simulink model "pattern3x3_testing_2023v1"  (R2023a)
settings: Solver=FixedStepAuto  StartTime=0.0  StopTime=2  FixedStep=0.000005  RelTol=1e-3
values from neighbouring files (symbols this model uses):
  test_pattern = load('Pattern4_test.CSV')    [model_setup_test.m]
  Th_control_time2 = 0.02    [model_setup4.m]    (also in model_setup_test.m = 2)
  Th_minus_count2 = 10    [model_setup4.m]    (also in model_setup_test.m = 5)
  Th_plus_count2 = 20    [model_setup4.m]    (also in model_setup_test.m)
libraries: simulink x1
(part 2 of 4)

== system pattern3x3_testing_2023v1/Synapse12 ==
  note: Synapse
  Pre_spike : Inport
  addr : Inport  Port=2
  From Workspace : FromWorkspace  VariableName=syna_var
  MATLAB Function1 : MATLAB Function  TreatAsAtomicUnit=on
  Memory2 : Memory
  Product : Product
  Spike_gererator : Subsystem
  Weight : Outport
  Spike_out : Outport  Port=2
  Weight_out : Outport  Port=3
  wires:
  MATLAB Function1/1(y) -> Weight_out/1, Product/2
  Spike_gererator/1(Spike_out) -> Spike_out/1, Product/1
  Product/1 -> Weight/1
  Pre_spike/1 -> Memory2/1
  From Workspace/1 -> MATLAB Function1/1(syna_var)
  addr/1 -> MATLAB Function1/2(addr)
  Memory2/1 -> Spike_gererator/1("Spike ")

== system pattern3x3_testing_2023v1/Synapse13 ==
  note: Synapse
  Pre_spike : Inport
  addr : Inport  Port=2
  From Workspace : FromWorkspace  VariableName=syna_var
  MATLAB Function1 : MATLAB Function  TreatAsAtomicUnit=on
  Memory2 : Memory
  Product : Product
  Spike_gererator : Subsystem
  Weight : Outport
  Spike_out : Outport  Port=2
  Weight_out : Outport  Port=3
  wires:
  MATLAB Function1/1(y) -> Weight_out/1, Product/2
  Spike_gererator/1(Spike_out) -> Spike_out/1, Product/1
  Product/1 -> Weight/1
  Pre_spike/1 -> Memory2/1
  From Workspace/1 -> MATLAB Function1/1(syna_var)
  addr/1 -> MATLAB Function1/2(addr)
  Memory2/1 -> Spike_gererator/1("Spike ")

== system pattern3x3_testing_2023v1/Synapse14 ==
  note: Synapse
  Pre_spike : Inport
  addr : Inport  Port=2
  From Workspace : FromWorkspace  VariableName=syna_var
  MATLAB Function1 : MATLAB Function  TreatAsAtomicUnit=on
  Memory2 : Memory
  Product : Product
  Spike_gererator : Subsystem
  Weight : Outport
  Spike_out : Outport  Port=2
  Weight_out : Outport  Port=3
  wires:
  MATLAB Function1/1(y) -> Weight_out/1, Product/2
  Spike_gererator/1(Spike_out) -> Spike_out/1, Product/1
  Product/1 -> Weight/1
  Pre_spike/1 -> Memory2/1
  From Workspace/1 -> MATLAB Function1/1(syna_var)
  addr/1 -> MATLAB Function1/2(addr)
  Memory2/1 -> Spike_gererator/1("Spike ")

== system pattern3x3_testing_2023v1/Synapse15 ==
  note: Synapse
  Pre_spike : Inport
  addr : Inport  Port=2
  From Workspace : FromWorkspace  VariableName=syna_var
  MATLAB Function1 : MATLAB Function  TreatAsAtomicUnit=on
  Memory2 : Memory
  Product : Product
  Spike_gererator : Subsystem
  Weight : Outport
  Spike_out : Outport  Port=2
  Weight_out : Outport  Port=3
  wires:
  MATLAB Function1/1(y) -> Weight_out/1, Product/2
  Spike_gererator/1(Spike_out) -> Spike_out/1, Product/1
  Product/1 -> Weight/1
  Pre_spike/1 -> Memory2/1
  From Workspace/1 -> MATLAB Function1/1(syna_var)
  addr/1 -> MATLAB Function1/2(addr)
  Memory2/1 -> Spike_gererator/1("Spike ")

== system pattern3x3_testing_2023v1/Synapse16 ==
  note: Synapse
  Pre_spike : Inport
  addr : Inport  Port=2
  From Workspace : FromWorkspace  VariableName=syna_var
  MATLAB Function1 : MATLAB Function  TreatAsAtomicUnit=on
  Memory2 : Memory
  Product : Product
  Spike_gererator : Subsystem
  Weight : Outport
  Spike_out : Outport  Port=2
  Weight_out : Outport  Port=3
  wires:
  MATLAB Function1/1(y) -> Weight_out/1, Product/2
  Spike_gererator/1(Spike_out) -> Spike_out/1, Product/1
  Product/1 -> Weight/1
  Pre_spike/1 -> Memory2/1
  From Workspace/1 -> MATLAB Function1/1(syna_var)
  addr/1 -> MATLAB Function1/2(addr)
  Memory2/1 -> Spike_gererator/1("Spike ")

== system pattern3x3_testing_2023v1/Synapse17 ==
  note: Synapse
  Pre_spike : Inport
  addr : Inport  Port=2
  From Workspace : FromWorkspace  VariableName=syna_var
  MATLAB Function1 : MATLAB Function  TreatAsAtomicUnit=on
  Memory2 : Memory
  Product : Product
  Spike_gererator : Subsystem
  Weight : Outport
  Spike_out : Outport  Port=2
  Weight_out : Outport  Port=3
  wires:
  MATLAB Function1/1(y) -> Weight_out/1, Product/2
  Spike_gererator/1(Spike_out) -> Spike_out/1, Product/1
  Product/1 -> Weight/1
  Pre_spike/1 -> Memory2/1
  From Workspace/1 -> MATLAB Function1/1(syna_var)
  addr/1 -> MATLAB Function1/2(addr)
  Memory2/1 -> Spike_gererator/1("Spike ")

== system pattern3x3_testing_2023v1/Synapse18 ==
  note: Synapse
  Pre_spike : Inport
  addr : Inport  Port=2
  From Workspace : FromWorkspace  VariableName=syna_var
  MATLAB Function1 : MATLAB Function  TreatAsAtomicUnit=on
  Memory2 : Memory
  Product : Product
  Spike_gererator : Subsystem
  Weight : Outport
  Spike_out : Outport  Port=2
  Weight_out : Outport  Port=3
  wires:
  MATLAB Function1/1(y) -> Weight_out/1, Product/2
  Spike_gererator/1(Spike_out) -> Spike_out/1, Product/1
  Product/1 -> Weight/1
  Pre_spike/1 -> Memory2/1
  From Workspace/1 -> MATLAB Function1/1(syna_var)
  addr/1 -> MATLAB Function1/2(addr)
  Memory2/1 -> Spike_gererator/1("Spike ")

== system pattern3x3_testing_2023v1/Synapse19 ==
  note: Synapse
  Pre_spike : Inport
  addr : Inport  Port=2
  From Workspace : FromWorkspace  VariableName=syna_var
  MATLAB Function1 : MATLAB Function  TreatAsAtomicUnit=on
  Memory2 : Memory
  Product : Product
  Spike_gererator : Subsystem
  Weight : Outport
  Spike_out : Outport  Port=2
  Weight_out : Outport  Port=3
  wires:
  MATLAB Function1/1(y) -> Weight_out/1, Product/2
  Spike_gererator/1(Spike_out) -> Spike_out/1, Product/1
  Product/1 -> Weight/1
  Pre_spike/1 -> Memory2/1
  From Workspace/1 -> MATLAB Function1/1(syna_var)
  addr/1 -> MATLAB Function1/2(addr)
  Memory2/1 -> Spike_gererator/1("Spike ")

== system pattern3x3_testing_2023v1/Synapse2 ==
  note: Synapse
  Pre_spike : Inport
  addr : Inport  Port=2
  From Workspace : FromWorkspace  VariableName=syna_var
  MATLAB Function1 : MATLAB Function  TreatAsAtomicUnit=on
  Memory2 : Memory
  Product : Product
  Spike_gererator : Subsystem
  Weight : Outport
  Spike_out : Outport  Port=2
  Weight_out : Outport  Port=3
  wires:
  MATLAB Function1/1(y) -> Weight_out/1, Product/2
  Spike_gererator/1(Spike_out) -> Spike_out/1, Product/1
  Product/1 -> Weight/1
  Pre_spike/1 -> Memory2/1
  From Workspace/1 -> MATLAB Function1/1(syna_var)
  addr/1 -> MATLAB Function1/2(addr)
  Memory2/1 -> Spike_gererator/1("Spike ")

== system pattern3x3_testing_2023v1/Synapse20 ==
  note: Synapse
  Pre_spike : Inport
  addr : Inport  Port=2
  From Workspace : FromWorkspace  VariableName=syna_var
  MATLAB Function1 : MATLAB Function  TreatAsAtomicUnit=on
  Memory2 : Memory
  Product : Product
  Spike_gererator : Subsystem
  Weight : Outport
  Spike_out : Outport  Port=2
  Weight_out : Outport  Port=3
  wires:
  MATLAB Function1/1(y) -> Weight_out/1, Product/2
  Spike_gererator/1(Spike_out) -> Spike_out/1, Product/1
  Product/1 -> Weight/1
  Pre_spike/1 -> Memory2/1
  From Workspace/1 -> MATLAB Function1/1(syna_var)
  addr/1 -> MATLAB Function1/2(addr)
  Memory2/1 -> Spike_gererator/1("Spike ")

== system pattern3x3_testing_2023v1/Synapse21 ==
  note: Synapse
  Pre_spike : Inport
  addr : Inport  Port=2
  From Workspace : FromWorkspace  VariableName=syna_var
  MATLAB Function1 : MATLAB Function  TreatAsAtomicUnit=on
  Memory2 : Memory
  Product : Product
  Spike_gererator : Subsystem
  Weight : Outport
  Spike_out : Outport  Port=2
  Weight_out : Outport  Port=3
  wires:
  MATLAB Function1/1(y) -> Weight_out/1, Product/2
  Spike_gererator/1(Spike_out) -> Spike_out/1, Product/1
  Product/1 -> Weight/1
  Pre_spike/1 -> Memory2/1
  From Workspace/1 -> MATLAB Function1/1(syna_var)
  addr/1 -> MATLAB Function1/2(addr)
  Memory2/1 -> Spike_gererator/1("Spike ")

== system pattern3x3_testing_2023v1/Synapse22 ==
  note: Synapse
  Pre_spike : Inport
  addr : Inport  Port=2
  From Workspace : FromWorkspace  VariableName=syna_var
  MATLAB Function1 : MATLAB Function  TreatAsAtomicUnit=on
  Memory2 : Memory
  Product : Product
  Spike_gererator : Subsystem
  Weight : Outport
  Spike_out : Outport  Port=2
  Weight_out : Outport  Port=3
  wires:
  MATLAB Function1/1(y) -> Weight_out/1, Product/2
  Spike_gererator/1(Spike_out) -> Spike_out/1, Product/1
  Product/1 -> Weight/1
  Pre_spike/1 -> Memory2/1
  From Workspace/1 -> MATLAB Function1/1(syna_var)
  addr/1 -> MATLAB Function1/2(addr)
  Memory2/1 -> Spike_gererator/1("Spike ")

== system pattern3x3_testing_2023v1/Synapse23 ==
  note: Synapse
  Pre_spike : Inport
  addr : Inport  Port=2
  From Workspace : FromWorkspace  VariableName=syna_var
  MATLAB Function1 : MATLAB Function  TreatAsAtomicUnit=on
  Memory2 : Memory
  Product : Product
  Spike_gererator : Subsystem
  Weight : Outport
  Spike_out : Outport  Port=2
  Weight_out : Outport  Port=3
  wires:
  MATLAB Function1/1(y) -> Weight_out/1, Product/2
  Spike_gererator/1(Spike_out) -> Spike_out/1, Product/1
  Product/1 -> Weight/1
  Pre_spike/1 -> Memory2/1
  From Workspace/1 -> MATLAB Function1/1(syna_var)
  addr/1 -> MATLAB Function1/2(addr)
  Memory2/1 -> Spike_gererator/1("Spike ")

== system pattern3x3_testing_2023v1/Synapse24 ==
  note: Synapse
  Pre_spike : Inport
  addr : Inport  Port=2
  From Workspace : FromWorkspace  VariableName=syna_var
  MATLAB Function1 : MATLAB Function  TreatAsAtomicUnit=on
  Memory2 : Memory
  Product : Product
  Spike_gererator : Subsystem
  Weight : Outport
  Spike_out : Outport  Port=2
  Weight_out : Outport  Port=3
  wires:
  MATLAB Function1/1(y) -> Weight_out/1, Product/2
  Spike_gererator/1(Spike_out) -> Spike_out/1, Product/1
  Product/1 -> Weight/1
  Pre_spike/1 -> Memory2/1
  From Workspace/1 -> MATLAB Function1/1(syna_var)
  addr/1 -> MATLAB Function1/2(addr)
  Memory2/1 -> Spike_gererator/1("Spike ")

== system pattern3x3_testing_2023v1/Synapse25 ==
  note: Synapse
  Pre_spike : Inport
  addr : Inport  Port=2
  From Workspace : FromWorkspace  VariableName=syna_var
  MATLAB Function1 : MATLAB Function  TreatAsAtomicUnit=on
  Memory2 : Memory
  Product : Product
  Spike_gererator : Subsystem
  Weight : Outport
  Spike_out : Outport  Port=2
  Weight_out : Outport  Port=3
  wires:
  MATLAB Function1/1(y) -> Weight_out/1, Product/2
  Spike_gererator/1(Spike_out) -> Spike_out/1, Product/1
  Product/1 -> Weight/1
  Pre_spike/1 -> Memory2/1
  From Workspace/1 -> MATLAB Function1/1(syna_var)
  addr/1 -> MATLAB Function1/2(addr)
  Memory2/1 -> Spike_gererator/1("Spike ")

== system pattern3x3_testing_2023v1/Synapse26 ==
  note: Synapse
  Pre_spike : Inport
  addr : Inport  Port=2
  From Workspace : FromWorkspace  VariableName=syna_var
  MATLAB Function1 : MATLAB Function  TreatAsAtomicUnit=on
  Memory2 : Memory
  Product : Product
  Spike_gererator : Subsystem
  Weight : Outport
  Spike_out : Outport  Port=2
  Weight_out : Outport  Port=3
  wires:
  MATLAB Function1/1(y) -> Weight_out/1, Product/2
  Spike_gererator/1(Spike_out) -> Spike_out/1, Product/1
  Product/1 -> Weight/1
  Pre_spike/1 -> Memory2/1
  From Workspace/1 -> MATLAB Function1/1(syna_var)
  addr/1 -> MATLAB Function1/2(addr)
  Memory2/1 -> Spike_gererator/1("Spike ")

== system pattern3x3_testing_2023v1/Synapse27 ==
  note: Synapse
  Pre_spike : Inport
  addr : Inport  Port=2
  From Workspace : FromWorkspace  VariableName=syna_var
  MATLAB Function1 : MATLAB Function  TreatAsAtomicUnit=on
  Memory2 : Memory
  Product : Product
  Spike_gererator : Subsystem
  Weight : Outport
  Spike_out : Outport  Port=2
  Weight_out : Outport  Port=3
  wires:
  MATLAB Function1/1(y) -> Weight_out/1, Product/2
  Spike_gererator/1(Spike_out) -> Spike_out/1, Product/1
  Product/1 -> Weight/1
  Pre_spike/1 -> Memory2/1
  From Workspace/1 -> MATLAB Function1/1(syna_var)
  addr/1 -> MATLAB Function1/2(addr)
  Memory2/1 -> Spike_gererator/1("Spike ")

== system pattern3x3_testing_2023v1/Synapse28 ==
  note: Synapse
  Pre_spike : Inport
  addr : Inport  Port=2
  From Workspace : FromWorkspace  VariableName=syna_var
  MATLAB Function1 : MATLAB Function  TreatAsAtomicUnit=on
  Memory2 : Memory
  Product : Product
  Spike_gererator : Subsystem
  Weight : Outport
  Spike_out : Outport  Port=2
  Weight_out : Outport  Port=3
  wires:
  MATLAB Function1/1(y) -> Weight_out/1, Product/2
  Spike_gererator/1(Spike_out) -> Spike_out/1, Product/1
  Product/1 -> Weight/1
  Pre_spike/1 -> Memory2/1
  From Workspace/1 -> MATLAB Function1/1(syna_var)
  addr/1 -> MATLAB Function1/2(addr)
  Memory2/1 -> Spike_gererator/1("Spike ")

== system pattern3x3_testing_2023v1/Synapse29 ==
  note: Synapse
  Pre_spike : Inport
  addr : Inport  Port=2
  From Workspace : FromWorkspace  VariableName=syna_var
  MATLAB Function1 : MATLAB Function  TreatAsAtomicUnit=on
  Memory2 : Memory
  Product : Product
  Spike_gererator : Subsystem
  Weight : Outport
  Spike_out : Outport  Port=2
  Weight_out : Outport  Port=3
  wires:
  MATLAB Function1/1(y) -> Weight_out/1, Product/2
  Spike_gererator/1(Spike_out) -> Spike_out/1, Product/1
  Product/1 -> Weight/1
  Pre_spike/1 -> Memory2/1
  From Workspace/1 -> MATLAB Function1/1(syna_var)
  addr/1 -> MATLAB Function1/2(addr)
  Memory2/1 -> Spike_gererator/1("Spike ")

== system pattern3x3_testing_2023v1/Synapse3 ==
  note: Synapse
  Pre_spike : Inport
  addr : Inport  Port=2
  From Workspace : FromWorkspace  VariableName=syna_var
  MATLAB Function1 : MATLAB Function  TreatAsAtomicUnit=on
  Memory2 : Memory
  Product : Product
  Spike_gererator : Subsystem
  Weight : Outport
  Spike_out : Outport  Port=2
  Weight_out : Outport  Port=3
  wires:
  MATLAB Function1/1(y) -> Weight_out/1, Product/2
  Spike_gererator/1(Spike_out) -> Spike_out/1, Product/1
  Product/1 -> Weight/1
  Pre_spike/1 -> Memory2/1
  From Workspace/1 -> MATLAB Function1/1(syna_var)
  addr/1 -> MATLAB Function1/2(addr)
  Memory2/1 -> Spike_gererator/1("Spike ")

== system pattern3x3_testing_2023v1/Synapse30 ==
  note: Synapse
  Pre_spike : Inport
  addr : Inport  Port=2
  From Workspace : FromWorkspace  VariableName=syna_var
  MATLAB Function1 : MATLAB Function  TreatAsAtomicUnit=on
  Memory2 : Memory
  Product : Product
  Spike_gererator : Subsystem
  Weight : Outport
  Spike_out : Outport  Port=2
  Weight_out : Outport  Port=3
  wires:
  MATLAB Function1/1(y) -> Weight_out/1, Product/2
  Spike_gererator/1(Spike_out) -> Spike_out/1, Product/1
  Product/1 -> Weight/1
  Pre_spike/1 -> Memory2/1
  From Workspace/1 -> MATLAB Function1/1(syna_var)
  addr/1 -> MATLAB Function1/2(addr)
  Memory2/1 -> Spike_gererator/1("Spike ")

== system pattern3x3_testing_2023v1/Synapse31 ==
  note: Synapse
  Pre_spike : Inport
  addr : Inport  Port=2
  From Workspace : FromWorkspace  VariableName=syna_var
  MATLAB Function1 : MATLAB Function  TreatAsAtomicUnit=on
  Memory2 : Memory
  Product : Product
  Spike_gererator : Subsystem
  Weight : Outport
  Spike_out : Outport  Port=2
  Weight_out : Outport  Port=3
  wires:
  MATLAB Function1/1(y) -> Weight_out/1, Product/2
  Spike_gererator/1(Spike_out) -> Spike_out/1, Product/1
  Product/1 -> Weight/1
  Pre_spike/1 -> Memory2/1
  From Workspace/1 -> MATLAB Function1/1(syna_var)
  addr/1 -> MATLAB Function1/2(addr)
  Memory2/1 -> Spike_gererator/1("Spike ")

== system pattern3x3_testing_2023v1/Synapse32 ==
  note: Synapse
  Pre_spike : Inport
  addr : Inport  Port=2
  From Workspace : FromWorkspace  VariableName=syna_var
  MATLAB Function1 : MATLAB Function  TreatAsAtomicUnit=on
  Memory2 : Memory
  Product : Product
  Spike_gererator : Subsystem
  Weight : Outport
  Spike_out : Outport  Port=2
  Weight_out : Outport  Port=3
  wires:
  MATLAB Function1/1(y) -> Weight_out/1, Product/2
  Spike_gererator/1(Spike_out) -> Spike_out/1, Product/1
  Product/1 -> Weight/1
  Pre_spike/1 -> Memory2/1
  From Workspace/1 -> MATLAB Function1/1(syna_var)
  addr/1 -> MATLAB Function1/2(addr)
  Memory2/1 -> Spike_gererator/1("Spike ")

== system pattern3x3_testing_2023v1/Synapse33 ==
  note: Synapse
  Pre_spike : Inport
  addr : Inport  Port=2
  From Workspace : FromWorkspace  VariableName=syna_var
  MATLAB Function1 : MATLAB Function  TreatAsAtomicUnit=on
  Memory2 : Memory
  Product : Product
  Spike_gererator : Subsystem
  Weight : Outport
  Spike_out : Outport  Port=2
  Weight_out : Outport  Port=3
  wires:
  MATLAB Function1/1(y) -> Weight_out/1, Product/2
  Spike_gererator/1(Spike_out) -> Spike_out/1, Product/1
  Product/1 -> Weight/1
  Pre_spike/1 -> Memory2/1
  From Workspace/1 -> MATLAB Function1/1(syna_var)
  addr/1 -> MATLAB Function1/2(addr)
  Memory2/1 -> Spike_gererator/1("Spike ")

== system pattern3x3_testing_2023v1/Synapse34 ==
  note: Synapse
  Pre_spike : Inport
  addr : Inport  Port=2
  From Workspace : FromWorkspace  VariableName=syna_var
  MATLAB Function1 : MATLAB Function  TreatAsAtomicUnit=on
  Memory2 : Memory
  Product : Product
  Spike_gererator : Subsystem
  Weight : Outport
  Spike_out : Outport  Port=2
  Weight_out : Outport  Port=3
  wires:
  MATLAB Function1/1(y) -> Weight_out/1, Product/2
  Spike_gererator/1(Spike_out) -> Spike_out/1, Product/1
  Product/1 -> Weight/1
  Pre_spike/1 -> Memory2/1
  From Workspace/1 -> MATLAB Function1/1(syna_var)
  addr/1 -> MATLAB Function1/2(addr)
  Memory2/1 -> Spike_gererator/1("Spike ")

== system pattern3x3_testing_2023v1/Synapse35 ==
  note: Synapse
  Pre_spike : Inport
  addr : Inport  Port=2
  From Workspace : FromWorkspace  VariableName=syna_var
  MATLAB Function1 : MATLAB Function  TreatAsAtomicUnit=on
  Memory2 : Memory
  Product : Product
  Spike_gererator : Subsystem
  Weight : Outport
  Spike_out : Outport  Port=2
  Weight_out : Outport  Port=3
  wires:
  MATLAB Function1/1(y) -> Weight_out/1, Product/2
  Spike_gererator/1(Spike_out) -> Spike_out/1, Product/1
  Product/1 -> Weight/1
  Pre_spike/1 -> Memory2/1
  From Workspace/1 -> MATLAB Function1/1(syna_var)
  addr/1 -> MATLAB Function1/2(addr)
  Memory2/1 -> Spike_gererator/1("Spike ")

== system pattern3x3_testing_2023v1/Synapse36 ==
  note: Synapse
  Pre_spike : Inport
  addr : Inport  Port=2
  From Workspace : FromWorkspace  VariableName=syna_var
  MATLAB Function1 : MATLAB Function  TreatAsAtomicUnit=on
  Memory2 : Memory
  Product : Product
  Spike_gererator : Subsystem
  Weight : Outport
  Spike_out : Outport  Port=2
  Weight_out : Outport  Port=3
  wires:
  MATLAB Function1/1(y) -> Weight_out/1, Product/2
  Spike_gererator/1(Spike_out) -> Spike_out/1, Product/1
  Product/1 -> Weight/1
  Pre_spike/1 -> Memory2/1
  From Workspace/1 -> MATLAB Function1/1(syna_var)
  addr/1 -> MATLAB Function1/2(addr)
  Memory2/1 -> Spike_gererator/1("Spike ")

== system pattern3x3_testing_2023v1/Synapse4 ==
  note: Synapse
  Pre_spike : Inport
  addr : Inport  Port=2
  From Workspace : FromWorkspace  VariableName=syna_var
  MATLAB Function1 : MATLAB Function  TreatAsAtomicUnit=on
  Memory2 : Memory
  Product : Product
  Spike_gererator : Subsystem
  Weight : Outport
  Spike_out : Outport  Port=2
  Weight_out : Outport  Port=3
  wires:
  MATLAB Function1/1(y) -> Weight_out/1, Product/2
  Spike_gererator/1(Spike_out) -> Spike_out/1, Product/1
  Product/1 -> Weight/1
  Pre_spike/1 -> Memory2/1
  From Workspace/1 -> MATLAB Function1/1(syna_var)
  addr/1 -> MATLAB Function1/2(addr)
  Memory2/1 -> Spike_gererator/1("Spike ")

== system pattern3x3_testing_2023v1/Synapse5 ==
  note: Synapse
  Pre_spike : Inport
  addr : Inport  Port=2
  From Workspace : FromWorkspace  VariableName=syna_var
  MATLAB Function1 : MATLAB Function  TreatAsAtomicUnit=on
  Memory2 : Memory
  Product : Product
  Spike_gererator : Subsystem
  Weight : Outport
  Spike_out : Outport  Port=2
  Weight_out : Outport  Port=3
  wires:
  MATLAB Function1/1(y) -> Weight_out/1, Product/2
  Spike_gererator/1(Spike_out) -> Spike_out/1, Product/1
  Product/1 -> Weight/1
  Pre_spike/1 -> Memory2/1
  From Workspace/1 -> MATLAB Function1/1(syna_var)
  addr/1 -> MATLAB Function1/2(addr)
  Memory2/1 -> Spike_gererator/1("Spike ")

== system pattern3x3_testing_2023v1/Synapse6 ==
  note: Synapse
  Pre_spike : Inport
  addr : Inport  Port=2
  From Workspace : FromWorkspace  VariableName=syna_var
  MATLAB Function1 : MATLAB Function  TreatAsAtomicUnit=on
  Memory2 : Memory
  Product : Product
  Spike_gererator : Subsystem
  Weight : Outport
  Spike_out : Outport  Port=2
  Weight_out : Outport  Port=3
  wires:
  MATLAB Function1/1(y) -> Weight_out/1, Product/2
  Spike_gererator/1(Spike_out) -> Spike_out/1, Product/1
  Product/1 -> Weight/1
  Pre_spike/1 -> Memory2/1
  From Workspace/1 -> MATLAB Function1/1(syna_var)
  addr/1 -> MATLAB Function1/2(addr)
  Memory2/1 -> Spike_gererator/1("Spike ")

== system pattern3x3_testing_2023v1/Synapse7 ==
  note: Synapse
  Pre_spike : Inport
  addr : Inport  Port=2
  From Workspace : FromWorkspace  VariableName=syna_var
  MATLAB Function1 : MATLAB Function  TreatAsAtomicUnit=on
  Memory2 : Memory
  Product : Product
  Spike_gererator : Subsystem
  Weight : Outport
  Spike_out : Outport  Port=2
  Weight_out : Outport  Port=3
  wires:
  MATLAB Function1/1(y) -> Weight_out/1, Product/2
  Spike_gererator/1(Spike_out) -> Spike_out/1, Product/1
  Product/1 -> Weight/1
  Pre_spike/1 -> Memory2/1
  From Workspace/1 -> MATLAB Function1/1(syna_var)
  addr/1 -> MATLAB Function1/2(addr)
  Memory2/1 -> Spike_gererator/1("Spike ")

== system pattern3x3_testing_2023v1/Synapse8 ==
  note: Synapse
  Pre_spike : Inport
  addr : Inport  Port=2
  From Workspace : FromWorkspace  VariableName=syna_var
  MATLAB Function1 : MATLAB Function  TreatAsAtomicUnit=on
  Memory2 : Memory
  Product : Product
  Spike_gererator : Subsystem
  Weight : Outport
  Spike_out : Outport  Port=2
  Weight_out : Outport  Port=3
  wires:
  MATLAB Function1/1(y) -> Weight_out/1, Product/2
  Spike_gererator/1(Spike_out) -> Spike_out/1, Product/1
  Product/1 -> Weight/1
  Pre_spike/1 -> Memory2/1
  From Workspace/1 -> MATLAB Function1/1(syna_var)
  addr/1 -> MATLAB Function1/2(addr)
  Memory2/1 -> Spike_gererator/1("Spike ")

== system pattern3x3_testing_2023v1/Synapse9 ==
  note: Synapse
  Pre_spike : Inport
  addr : Inport  Port=2
  From Workspace : FromWorkspace  VariableName=syna_var
  MATLAB Function1 : MATLAB Function  TreatAsAtomicUnit=on
  Memory2 : Memory
  Product : Product
  Spike_gererator : Subsystem
  Weight : Outport
  Spike_out : Outport  Port=2
  Weight_out : Outport  Port=3
  wires:
  MATLAB Function1/1(y) -> Weight_out/1, Product/2
  Spike_gererator/1(Spike_out) -> Spike_out/1, Product/1
  Product/1 -> Weight/1
  Pre_spike/1 -> Memory2/1
  From Workspace/1 -> MATLAB Function1/1(syna_var)
  addr/1 -> MATLAB Function1/2(addr)
  Memory2/1 -> Spike_gererator/1("Spike ")

== system pattern3x3_testing_2023v1/Neuron1/Clock4 ==
  "Reset " : Inport
  Memory2 : Memory
  NOT1 : Logic  Operator=NOT  IconShape=distinctive  AllPortsSameDT=off  OutDataTypeStr=boolean
  Product1 : Product
  Pulse Generator1 : DiscretePulseGenerator  PulseType=Time based  Period=0.00001  PulseWidth=50
  Triggered Subsystem1 : Subsystem  TreatAsAtomicUnit=on
  T : Outport  VectorParamsAs1DForOutWhenUnconnected=off
  wires:
  Memory2/1 -> Triggered Subsystem1/1(In1)
  Product1/1 -> T/1, Memory2/1
  Pulse Generator1/1 -> Triggered Subsystem1/Trigger
  "Reset "/1 -> NOT1/1
  Triggered Subsystem1/1(Out1) -> Product1/1
  NOT1/1 -> Product1/2

== system pattern3x3_testing_2023v1/Neuron1/Clock5 ==
  "Reset " : Inport
  Memory2 : Memory
  NOT1 : Logic  Operator=NOT  IconShape=distinctive  AllPortsSameDT=off  OutDataTypeStr=boolean
  Product1 : Product
  Pulse Generator1 : DiscretePulseGenerator  PulseType=Time based  Period=0.00001  PulseWidth=50
  Triggered Subsystem1 : Subsystem  TreatAsAtomicUnit=on
  T : Outport  VectorParamsAs1DForOutWhenUnconnected=off
  wires:
  Memory2/1 -> Triggered Subsystem1/1(In1)
  Product1/1 -> T/1, Memory2/1
  Pulse Generator1/1 -> Triggered Subsystem1/Trigger
  "Reset "/1 -> NOT1/1
  Triggered Subsystem1/1(Out1) -> Product1/1
  NOT1/1 -> Product1/2

== system pattern3x3_testing_2023v1/Neuron1/Subsystem2 ==
  note: 기존 membrane potential + input potential
  Input potential : Inport
  before_Potential : Inport  Port=2
  Trigger : TriggerPort  VariantControl=(inherit)  PortDimensions=1
  Sum : Sum  Inputs=|++
  membrane_state : Outport
  wires:
  Input potential/1 -> Sum/1
  Sum/1 -> membrane_state/1
  before_Potential/1 -> Sum/2

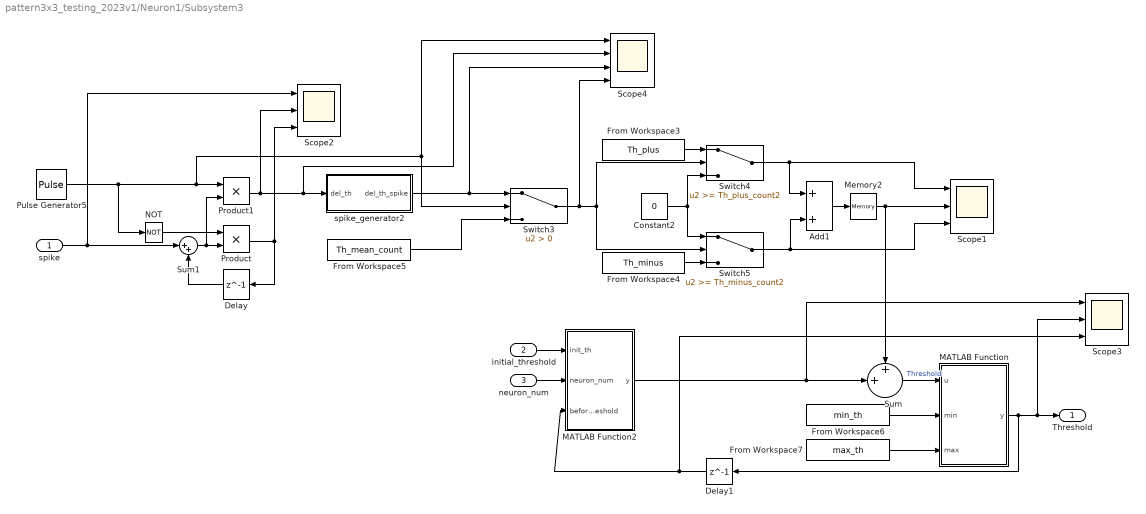
== system pattern3x3_testing_2023v1/Neuron1/Subsystem3 ==
  spike : Inport  OutDataTypeStr=double
  initial_threshold : Inport  Port=2
  neuron_num : Inport  Port=3
  Add1 : Sum
  Constant2 : Constant  Value=0
  Delay : Delay  DelayLength=1  SampleTime=0.00001
  Delay1 : Delay  DelayLength=1  SampleTime=0.00001
  From Workspace3 : FromWorkspace  VariableName=Th_plus
  From Workspace4 : FromWorkspace  VariableName=Th_minus
  From Workspace5 : FromWorkspace  VariableName=Th_mean_count
  From Workspace6 : FromWorkspace  VariableName=min_th
  From Workspace7 : FromWorkspace  VariableName=max_th
  MATLAB Function : MATLAB Function  TreatAsAtomicUnit=on
  MATLAB Function2 : MATLAB Function  TreatAsAtomicUnit=on
  Memory2 : Memory
  NOT : Logic  Operator=NOT  IconShape=distinctive  AllPortsSameDT=off  OutDataTypeStr=boolean
  Product : Product
  Product1 : Product
  Pulse Generator5 : DiscretePulseGenerator  PulseType=Time based  Period=Th_control_time2  PulseWidth=0.00001/Th_control_time2*100  PhaseDelay=Th_control_time2
  Scope1 : Scope  NumInputPorts=3
  Scope2 : Scope  NumInputPorts=3
  Scope3 : Scope  NumInputPorts=3
  Scope4 : Scope  NumInputPorts=4
  Sum : Sum  Inputs=++|
  Sum1 : Sum  Inputs=|++
  Switch3 : Switch  Criteria=u2 > Threshold  SaturateOnIntegerOverflow=off  InputSameDT=off
  Switch4 : Switch  Threshold=Th_plus_count2  SaturateOnIntegerOverflow=off  InputSameDT=off
  Switch5 : Switch  Threshold=Th_minus_count2  SaturateOnIntegerOverflow=off  InputSameDT=off
  spike_generator2 : Subsystem
  Threshold : Outport
  wires:
  MATLAB Function2/1(y) -> Scope3/1, Sum/2
  Sum/1 -> MATLAB Function/1(u)  "Threshold"
  From Workspace7/1 -> MATLAB Function/3(max)
  Delay1/1 -> Scope3/3, MATLAB Function2/3(before_threshold)
  neuron_num/1 -> MATLAB Function2/2(neuron_num)
  MATLAB Function/1(y) -> Delay1/1, Scope3/2, Threshold/1
  initial_threshold/1 -> MATLAB Function2/1(init_th)
  From Workspace6/1 -> MATLAB Function/2(min)
  Pulse Generator5/1 -> Switch3/2, Scope4/1, Product1/1, NOT/1
  Product1/1 -> Scope2/2, Scope4/2, spike_generator2/1(del_th)
  spike/1 -> Scope2/1, Sum1/1
  Delay/1 -> Sum1/2
  Product/1 -> Delay/1, Scope2/3
  Switch4/1 -> Add1/1, Scope1/1
  Switch5/1 -> Scope1/3, Add1/2
  Sum1/1 -> Product1/2, Product/2
  Constant2/1 -> Switch5/1, Switch4/3
  From Workspace4/1 -> Switch5/3
  Switch3/1 -> Scope4/4, Switch5/2, Switch4/2
  From Workspace3/1 -> Switch4/1
  NOT/1 -> Product/1
  spike_generator2/1(del_th_spike) -> Switch3/1, Scope4/3
  From Workspace5/1 -> Switch3/3
  Memory2/1 -> Scope1/2, Sum/1
  Add1/1 -> Memory2/1

== system pattern3x3_testing_2023v1/Neuron1/spike_generator1 ==
  1 : Inport
  AND : Logic  IconShape=distinctive  AllPortsSameDT=off  OutDataTypeStr=boolean
  Cast To Double : DataTypeConversion  OutDataTypeStr=double  SaturateOnIntegerOverflow=off  RndMeth=Floor
  Delay1 : Delay
  NOT : Logic  Operator=NOT  IconShape=distinctive  AllPortsSameDT=off  OutDataTypeStr=boolean
  Scope3 : Scope  NumInputPorts=5
  spike : Outport
  wires:
  NOT/1 -> Scope3/2, Delay1/1
  Delay1/1 -> Scope3/3, AND/2
  AND/1 -> Scope3/4, Cast To Double/1
  1/1 -> AND/1, Scope3/1, NOT/1
  Cast To Double/1 -> Scope3/5, spike/1

== system pattern3x3_testing_2023v1/Neuron2/Clock4 ==
  "Reset " : Inport
  Memory2 : Memory
  NOT1 : Logic  Operator=NOT  IconShape=distinctive  AllPortsSameDT=off  OutDataTypeStr=boolean
  Product1 : Product
  Pulse Generator1 : DiscretePulseGenerator  PulseType=Time based  Period=0.00001  PulseWidth=50
  Triggered Subsystem1 : Subsystem  TreatAsAtomicUnit=on
  T : Outport  VectorParamsAs1DForOutWhenUnconnected=off
  wires:
  Memory2/1 -> Triggered Subsystem1/1(In1)
  Product1/1 -> T/1, Memory2/1
  Pulse Generator1/1 -> Triggered Subsystem1/Trigger
  "Reset "/1 -> NOT1/1
  Triggered Subsystem1/1(Out1) -> Product1/1
  NOT1/1 -> Product1/2

== system pattern3x3_testing_2023v1/Neuron2/Clock5 ==
  "Reset " : Inport
  Memory2 : Memory
  NOT1 : Logic  Operator=NOT  IconShape=distinctive  AllPortsSameDT=off  OutDataTypeStr=boolean
  Product1 : Product
  Pulse Generator1 : DiscretePulseGenerator  PulseType=Time based  Period=0.00001  PulseWidth=50
  Triggered Subsystem1 : Subsystem  TreatAsAtomicUnit=on
  T : Outport  VectorParamsAs1DForOutWhenUnconnected=off
  wires:
  Memory2/1 -> Triggered Subsystem1/1(In1)
  Product1/1 -> T/1, Memory2/1
  Pulse Generator1/1 -> Triggered Subsystem1/Trigger
  "Reset "/1 -> NOT1/1
  Triggered Subsystem1/1(Out1) -> Product1/1
  NOT1/1 -> Product1/2

== system pattern3x3_testing_2023v1/Neuron2/Subsystem2 ==
  note: 기존 membrane potential + input potential
  Input potential : Inport
  before_Potential : Inport  Port=2
  Trigger : TriggerPort  VariantControl=(inherit)  PortDimensions=1
  Sum : Sum  Inputs=|++
  membrane_state : Outport
  wires:
  Input potential/1 -> Sum/1
  Sum/1 -> membrane_state/1
  before_Potential/1 -> Sum/2

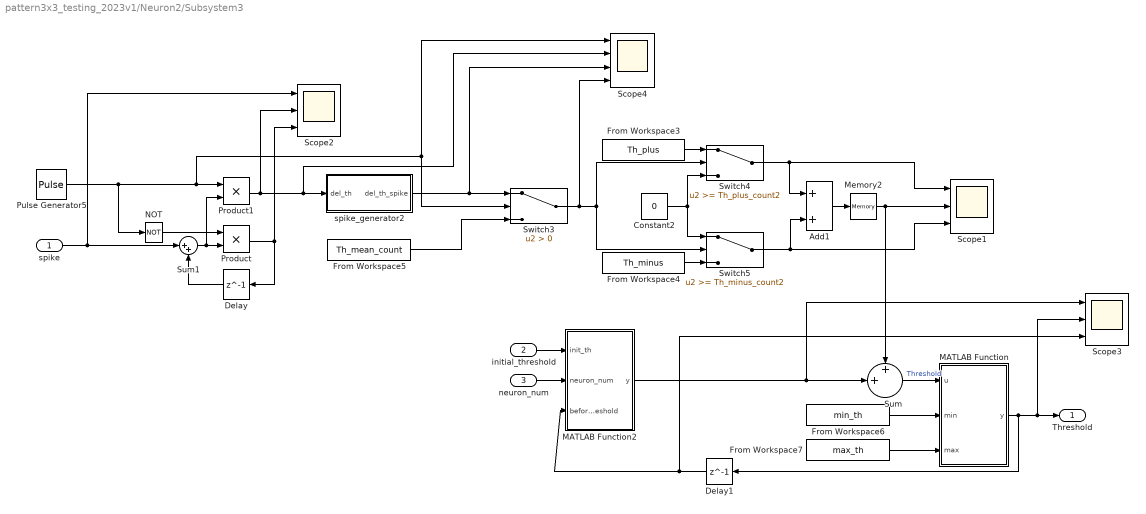
== system pattern3x3_testing_2023v1/Neuron2/Subsystem3 ==
  spike : Inport  OutDataTypeStr=double
  initial_threshold : Inport  Port=2
  neuron_num : Inport  Port=3
  Add1 : Sum
  Constant2 : Constant  Value=0
  Delay : Delay  DelayLength=1  SampleTime=0.00001
  Delay1 : Delay  DelayLength=1  SampleTime=0.00001
  From Workspace3 : FromWorkspace  VariableName=Th_plus
  From Workspace4 : FromWorkspace  VariableName=Th_minus
  From Workspace5 : FromWorkspace  VariableName=Th_mean_count
  From Workspace6 : FromWorkspace  VariableName=min_th
  From Workspace7 : FromWorkspace  VariableName=max_th
  MATLAB Function : MATLAB Function  TreatAsAtomicUnit=on
  MATLAB Function2 : MATLAB Function  TreatAsAtomicUnit=on
  Memory2 : Memory
  NOT : Logic  Operator=NOT  IconShape=distinctive  AllPortsSameDT=off  OutDataTypeStr=boolean
  Product : Product
  Product1 : Product
  Pulse Generator5 : DiscretePulseGenerator  PulseType=Time based  Period=Th_control_time2  PulseWidth=0.00001/Th_control_time2*100  PhaseDelay=Th_control_time2
  Scope1 : Scope  NumInputPorts=3
  Scope2 : Scope  NumInputPorts=3
  Scope3 : Scope  NumInputPorts=3
  Scope4 : Scope  NumInputPorts=4
  Sum : Sum  Inputs=++|
  Sum1 : Sum  Inputs=|++
  Switch3 : Switch  Criteria=u2 > Threshold  SaturateOnIntegerOverflow=off  InputSameDT=off
  Switch4 : Switch  Threshold=Th_plus_count2  SaturateOnIntegerOverflow=off  InputSameDT=off
  Switch5 : Switch  Threshold=Th_minus_count2  SaturateOnIntegerOverflow=off  InputSameDT=off
  spike_generator2 : Subsystem
  Threshold : Outport
  wires:
  MATLAB Function2/1(y) -> Scope3/1, Sum/2
  Sum/1 -> MATLAB Function/1(u)  "Threshold"
  From Workspace7/1 -> MATLAB Function/3(max)
  Delay1/1 -> Scope3/3, MATLAB Function2/3(before_threshold)
  neuron_num/1 -> MATLAB Function2/2(neuron_num)
  MATLAB Function/1(y) -> Delay1/1, Scope3/2, Threshold/1
  initial_threshold/1 -> MATLAB Function2/1(init_th)
  From Workspace6/1 -> MATLAB Function/2(min)
  Pulse Generator5/1 -> Switch3/2, Scope4/1, Product1/1, NOT/1
  Product1/1 -> Scope2/2, Scope4/2, spike_generator2/1(del_th)
  spike/1 -> Scope2/1, Sum1/1
  Delay/1 -> Sum1/2
  Product/1 -> Delay/1, Scope2/3
  Switch4/1 -> Add1/1, Scope1/1
  Switch5/1 -> Scope1/3, Add1/2
  Sum1/1 -> Product1/2, Product/2
  Constant2/1 -> Switch5/1, Switch4/3
  From Workspace4/1 -> Switch5/3
  Switch3/1 -> Scope4/4, Switch5/2, Switch4/2
  From Workspace3/1 -> Switch4/1
  NOT/1 -> Product/1
  spike_generator2/1(del_th_spike) -> Switch3/1, Scope4/3
  From Workspace5/1 -> Switch3/3
  Memory2/1 -> Scope1/2, Sum/1
  Add1/1 -> Memory2/1

== system pattern3x3_testing_2023v1/Neuron2/spike_generator1 ==
  1 : Inport
  AND : Logic  IconShape=distinctive  AllPortsSameDT=off  OutDataTypeStr=boolean
  Cast To Double : DataTypeConversion  OutDataTypeStr=double  SaturateOnIntegerOverflow=off  RndMeth=Floor
  Delay1 : Delay
  NOT : Logic  Operator=NOT  IconShape=distinctive  AllPortsSameDT=off  OutDataTypeStr=boolean
  Scope3 : Scope  NumInputPorts=5
  spike : Outport
  wires:
  NOT/1 -> Scope3/2, Delay1/1
  Delay1/1 -> Scope3/3, AND/2
  AND/1 -> Scope3/4, Cast To Double/1
  1/1 -> AND/1, Scope3/1, NOT/1
  Cast To Double/1 -> Scope3/5, spike/1

== system pattern3x3_testing_2023v1/Neuron3/Clock4 ==
  "Reset " : Inport
  Memory2 : Memory
  NOT1 : Logic  Operator=NOT  IconShape=distinctive  AllPortsSameDT=off  OutDataTypeStr=boolean
  Product1 : Product
  Pulse Generator1 : DiscretePulseGenerator  PulseType=Time based  Period=0.00001  PulseWidth=50
  Triggered Subsystem1 : Subsystem  TreatAsAtomicUnit=on
  T : Outport  VectorParamsAs1DForOutWhenUnconnected=off
  wires:
  Memory2/1 -> Triggered Subsystem1/1(In1)
  Product1/1 -> T/1, Memory2/1
  Pulse Generator1/1 -> Triggered Subsystem1/Trigger
  "Reset "/1 -> NOT1/1
  Triggered Subsystem1/1(Out1) -> Product1/1
  NOT1/1 -> Product1/2

== system pattern3x3_testing_2023v1/Neuron3/Clock5 ==
  "Reset " : Inport
  Memory2 : Memory
  NOT1 : Logic  Operator=NOT  IconShape=distinctive  AllPortsSameDT=off  OutDataTypeStr=boolean
  Product1 : Product
  Pulse Generator1 : DiscretePulseGenerator  PulseType=Time based  Period=0.00001  PulseWidth=50
  Triggered Subsystem1 : Subsystem  TreatAsAtomicUnit=on
  T : Outport  VectorParamsAs1DForOutWhenUnconnected=off
  wires:
  Memory2/1 -> Triggered Subsystem1/1(In1)
  Product1/1 -> T/1, Memory2/1
  Pulse Generator1/1 -> Triggered Subsystem1/Trigger
  "Reset "/1 -> NOT1/1
  Triggered Subsystem1/1(Out1) -> Product1/1
  NOT1/1 -> Product1/2

== system pattern3x3_testing_2023v1/Neuron3/Subsystem2 ==
  note: 기존 membrane potential + input potential
  Input potential : Inport
  before_Potential : Inport  Port=2
  Trigger : TriggerPort  VariantControl=(inherit)  PortDimensions=1
  Sum : Sum  Inputs=|++
  membrane_state : Outport
  wires:
  Input potential/1 -> Sum/1
  Sum/1 -> membrane_state/1
  before_Potential/1 -> Sum/2

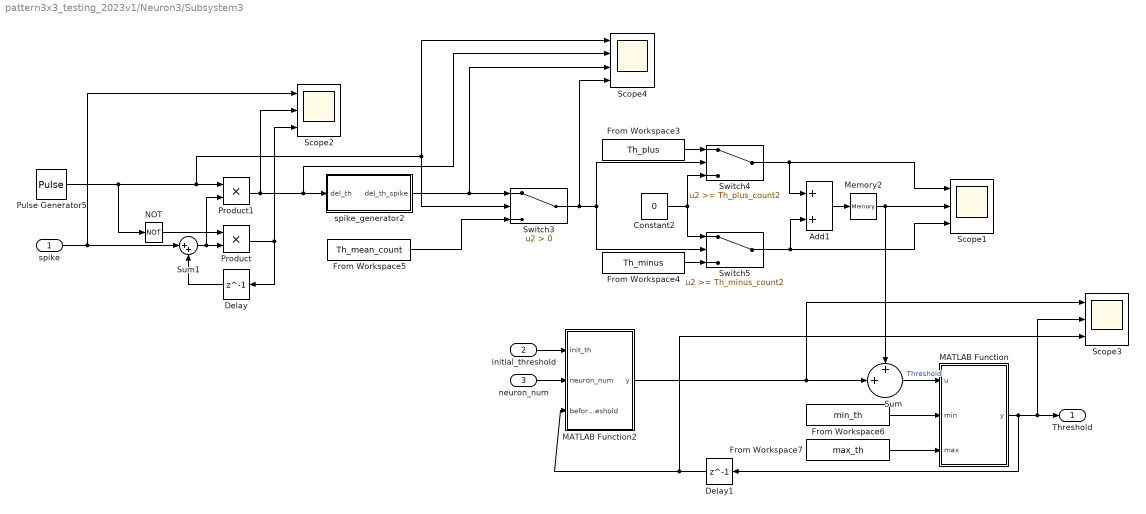
== system pattern3x3_testing_2023v1/Neuron3/Subsystem3 ==
  spike : Inport  OutDataTypeStr=double
  initial_threshold : Inport  Port=2
  neuron_num : Inport  Port=3
  Add1 : Sum
  Constant2 : Constant  Value=0
  Delay : Delay  DelayLength=1  SampleTime=0.00001
  Delay1 : Delay  DelayLength=1  SampleTime=0.00001
  From Workspace3 : FromWorkspace  VariableName=Th_plus
  From Workspace4 : FromWorkspace  VariableName=Th_minus
  From Workspace5 : FromWorkspace  VariableName=Th_mean_count
  From Workspace6 : FromWorkspace  VariableName=min_th
  From Workspace7 : FromWorkspace  VariableName=max_th
  MATLAB Function : MATLAB Function  TreatAsAtomicUnit=on
  MATLAB Function2 : MATLAB Function  TreatAsAtomicUnit=on
  Memory2 : Memory
  NOT : Logic  Operator=NOT  IconShape=distinctive  AllPortsSameDT=off  OutDataTypeStr=boolean
  Product : Product
  Product1 : Product
  Pulse Generator5 : DiscretePulseGenerator  PulseType=Time based  Period=Th_control_time2  PulseWidth=0.00001/Th_control_time2*100  PhaseDelay=Th_control_time2
  Scope1 : Scope  NumInputPorts=3
  Scope2 : Scope  NumInputPorts=3
  Scope3 : Scope  NumInputPorts=3
  Scope4 : Scope  NumInputPorts=4
  Sum : Sum  Inputs=++|
  Sum1 : Sum  Inputs=|++
  Switch3 : Switch  Criteria=u2 > Threshold  SaturateOnIntegerOverflow=off  InputSameDT=off
  Switch4 : Switch  Threshold=Th_plus_count2  SaturateOnIntegerOverflow=off  InputSameDT=off
  Switch5 : Switch  Threshold=Th_minus_count2  SaturateOnIntegerOverflow=off  InputSameDT=off
  spike_generator2 : Subsystem
  Threshold : Outport
  wires:
  MATLAB Function2/1(y) -> Scope3/1, Sum/2
  Sum/1 -> MATLAB Function/1(u)  "Threshold"
  From Workspace7/1 -> MATLAB Function/3(max)
  Delay1/1 -> Scope3/3, MATLAB Function2/3(before_threshold)
  neuron_num/1 -> MATLAB Function2/2(neuron_num)
  MATLAB Function/1(y) -> Delay1/1, Scope3/2, Threshold/1
  initial_threshold/1 -> MATLAB Function2/1(init_th)
  From Workspace6/1 -> MATLAB Function/2(min)
  Pulse Generator5/1 -> Switch3/2, Scope4/1, Product1/1, NOT/1
  Product1/1 -> Scope2/2, Scope4/2, spike_generator2/1(del_th)
  spike/1 -> Scope2/1, Sum1/1
  Delay/1 -> Sum1/2
  Product/1 -> Delay/1, Scope2/3
  Switch4/1 -> Add1/1, Scope1/1
  Switch5/1 -> Scope1/3, Add1/2
  Sum1/1 -> Product1/2, Product/2
  Constant2/1 -> Switch5/1, Switch4/3
  From Workspace4/1 -> Switch5/3
  Switch3/1 -> Scope4/4, Switch5/2, Switch4/2
  From Workspace3/1 -> Switch4/1
  NOT/1 -> Product/1
  spike_generator2/1(del_th_spike) -> Switch3/1, Scope4/3
  From Workspace5/1 -> Switch3/3
  Memory2/1 -> Scope1/2, Sum/1
  Add1/1 -> Memory2/1

== system pattern3x3_testing_2023v1/Neuron3/spike_generator1 ==
  1 : Inport
  AND : Logic  IconShape=distinctive  AllPortsSameDT=off  OutDataTypeStr=boolean
  Cast To Double : DataTypeConversion  OutDataTypeStr=double  SaturateOnIntegerOverflow=off  RndMeth=Floor
  Delay1 : Delay
  NOT : Logic  Operator=NOT  IconShape=distinctive  AllPortsSameDT=off  OutDataTypeStr=boolean
  Scope3 : Scope  NumInputPorts=5
  spike : Outport
  wires:
  NOT/1 -> Scope3/2, Delay1/1
  Delay1/1 -> Scope3/3, AND/2
  AND/1 -> Scope3/4, Cast To Double/1
  1/1 -> AND/1, Scope3/1, NOT/1
  Cast To Double/1 -> Scope3/5, spike/1

== system pattern3x3_testing_2023v1/Neuron4/Clock4 ==
  "Reset " : Inport
  Memory2 : Memory
  NOT1 : Logic  Operator=NOT  IconShape=distinctive  AllPortsSameDT=off  OutDataTypeStr=boolean
  Product1 : Product
  Pulse Generator1 : DiscretePulseGenerator  PulseType=Time based  Period=0.00001  PulseWidth=50
  Triggered Subsystem1 : Subsystem  TreatAsAtomicUnit=on
  T : Outport  VectorParamsAs1DForOutWhenUnconnected=off
  wires:
  Memory2/1 -> Triggered Subsystem1/1(In1)
  Product1/1 -> T/1, Memory2/1
  Pulse Generator1/1 -> Triggered Subsystem1/Trigger
  "Reset "/1 -> NOT1/1
  Triggered Subsystem1/1(Out1) -> Product1/1
  NOT1/1 -> Product1/2

== system pattern3x3_testing_2023v1/Neuron4/Clock5 ==
  "Reset " : Inport
  Memory2 : Memory
  NOT1 : Logic  Operator=NOT  IconShape=distinctive  AllPortsSameDT=off  OutDataTypeStr=boolean
  Product1 : Product
  Pulse Generator1 : DiscretePulseGenerator  PulseType=Time based  Period=0.00001  PulseWidth=50
  Triggered Subsystem1 : Subsystem  TreatAsAtomicUnit=on
  T : Outport  VectorParamsAs1DForOutWhenUnconnected=off
  wires:
  Memory2/1 -> Triggered Subsystem1/1(In1)
  Product1/1 -> T/1, Memory2/1
  Pulse Generator1/1 -> Triggered Subsystem1/Trigger
  "Reset "/1 -> NOT1/1
  Triggered Subsystem1/1(Out1) -> Product1/1
  NOT1/1 -> Product1/2

== system pattern3x3_testing_2023v1/Neuron4/Subsystem2 ==
  note: 기존 membrane potential + input potential
  Input potential : Inport
  before_Potential : Inport  Port=2
  Trigger : TriggerPort  VariantControl=(inherit)  PortDimensions=1
  Sum : Sum  Inputs=|++
  membrane_state : Outport
  wires:
  Input potential/1 -> Sum/1
  Sum/1 -> membrane_state/1
  before_Potential/1 -> Sum/2

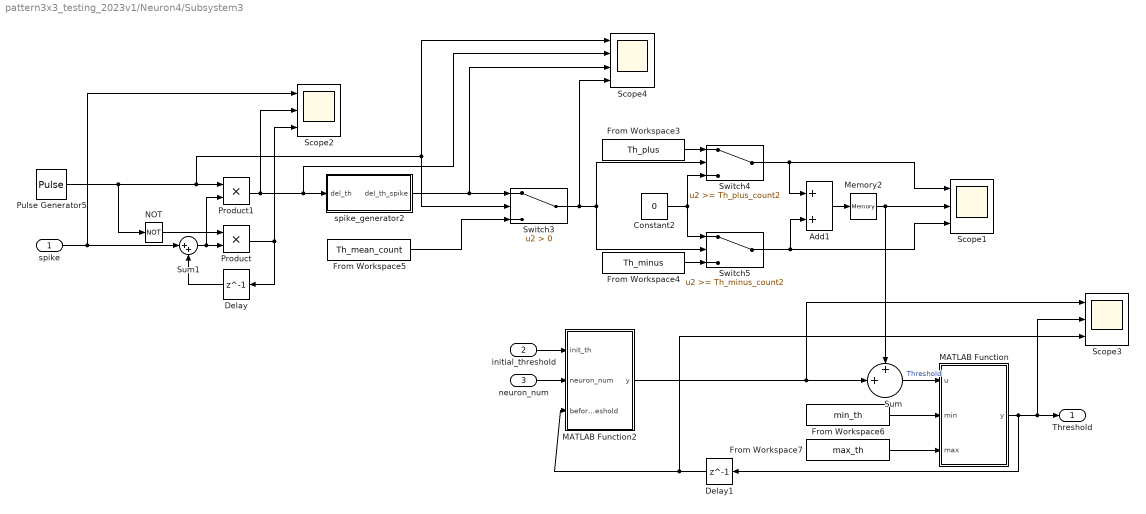
== system pattern3x3_testing_2023v1/Neuron4/Subsystem3 ==
  spike : Inport  OutDataTypeStr=double
  initial_threshold : Inport  Port=2
  neuron_num : Inport  Port=3
  Add1 : Sum
  Constant2 : Constant  Value=0
  Delay : Delay  DelayLength=1  SampleTime=0.00001
  Delay1 : Delay  DelayLength=1  SampleTime=0.00001
  From Workspace3 : FromWorkspace  VariableName=Th_plus
  From Workspace4 : FromWorkspace  VariableName=Th_minus
  From Workspace5 : FromWorkspace  VariableName=Th_mean_count
  From Workspace6 : FromWorkspace  VariableName=min_th
  From Workspace7 : FromWorkspace  VariableName=max_th
  MATLAB Function : MATLAB Function  TreatAsAtomicUnit=on
  MATLAB Function2 : MATLAB Function  TreatAsAtomicUnit=on
  Memory2 : Memory
  NOT : Logic  Operator=NOT  IconShape=distinctive  AllPortsSameDT=off  OutDataTypeStr=boolean
  Product : Product
  Product1 : Product
  Pulse Generator5 : DiscretePulseGenerator  PulseType=Time based  Period=Th_control_time2  PulseWidth=0.00001/Th_control_time2*100  PhaseDelay=Th_control_time2
  Scope1 : Scope  NumInputPorts=3
  Scope2 : Scope  NumInputPorts=3
  Scope3 : Scope  NumInputPorts=3
  Scope4 : Scope  NumInputPorts=4
  Sum : Sum  Inputs=++|
  Sum1 : Sum  Inputs=|++
  Switch3 : Switch  Criteria=u2 > Threshold  SaturateOnIntegerOverflow=off  InputSameDT=off
  Switch4 : Switch  Threshold=Th_plus_count2  SaturateOnIntegerOverflow=off  InputSameDT=off
  Switch5 : Switch  Threshold=Th_minus_count2  SaturateOnIntegerOverflow=off  InputSameDT=off
  spike_generator2 : Subsystem
  Threshold : Outport
  wires:
  MATLAB Function2/1(y) -> Scope3/1, Sum/2
  Sum/1 -> MATLAB Function/1(u)  "Threshold"
  From Workspace7/1 -> MATLAB Function/3(max)
  Delay1/1 -> Scope3/3, MATLAB Function2/3(before_threshold)
  neuron_num/1 -> MATLAB Function2/2(neuron_num)
  MATLAB Function/1(y) -> Delay1/1, Scope3/2, Threshold/1
  initial_threshold/1 -> MATLAB Function2/1(init_th)
  From Workspace6/1 -> MATLAB Function/2(min)
  Pulse Generator5/1 -> Switch3/2, Scope4/1, Product1/1, NOT/1
  Product1/1 -> Scope2/2, Scope4/2, spike_generator2/1(del_th)
  spike/1 -> Scope2/1, Sum1/1
  Delay/1 -> Sum1/2
  Product/1 -> Delay/1, Scope2/3
  Switch4/1 -> Add1/1, Scope1/1
  Switch5/1 -> Scope1/3, Add1/2
  Sum1/1 -> Product1/2, Product/2
  Constant2/1 -> Switch5/1, Switch4/3
  From Workspace4/1 -> Switch5/3
  Switch3/1 -> Scope4/4, Switch5/2, Switch4/2
  From Workspace3/1 -> Switch4/1
  NOT/1 -> Product/1
  spike_generator2/1(del_th_spike) -> Switch3/1, Scope4/3
  From Workspace5/1 -> Switch3/3
  Memory2/1 -> Scope1/2, Sum/1
  Add1/1 -> Memory2/1

== system pattern3x3_testing_2023v1/Neuron4/spike_generator1 ==
  1 : Inport
  AND : Logic  IconShape=distinctive  AllPortsSameDT=off  OutDataTypeStr=boolean
  Cast To Double : DataTypeConversion  OutDataTypeStr=double  SaturateOnIntegerOverflow=off  RndMeth=Floor
  Delay1 : Delay
  NOT : Logic  Operator=NOT  IconShape=distinctive  AllPortsSameDT=off  OutDataTypeStr=boolean
  Scope3 : Scope  NumInputPorts=5
  spike : Outport
  wires:
  NOT/1 -> Scope3/2, Delay1/1
  Delay1/1 -> Scope3/3, AND/2
  AND/1 -> Scope3/4, Cast To Double/1
  1/1 -> AND/1, Scope3/1, NOT/1
  Cast To Double/1 -> Scope3/5, spike/1

== system pattern3x3_testing_2023v1/Neuron5/Clock4 ==
  "Reset " : Inport
  Memory2 : Memory
  NOT1 : Logic  Operator=NOT  IconShape=distinctive  AllPortsSameDT=off  OutDataTypeStr=boolean
  Product1 : Product
  Pulse Generator1 : DiscretePulseGenerator  PulseType=Time based  Period=0.00001  PulseWidth=50
  Triggered Subsystem1 : Subsystem  TreatAsAtomicUnit=on
  T : Outport  VectorParamsAs1DForOutWhenUnconnected=off
  wires:
  Memory2/1 -> Triggered Subsystem1/1(In1)
  Product1/1 -> T/1, Memory2/1
  Pulse Generator1/1 -> Triggered Subsystem1/Trigger
  "Reset "/1 -> NOT1/1
  Triggered Subsystem1/1(Out1) -> Product1/1
  NOT1/1 -> Product1/2

== system pattern3x3_testing_2023v1/Neuron5/Clock5 ==
  "Reset " : Inport
  Memory2 : Memory
  NOT1 : Logic  Operator=NOT  IconShape=distinctive  AllPortsSameDT=off  OutDataTypeStr=boolean
  Product1 : Product
  Pulse Generator1 : DiscretePulseGenerator  PulseType=Time based  Period=0.00001  PulseWidth=50
  Triggered Subsystem1 : Subsystem  TreatAsAtomicUnit=on
  T : Outport  VectorParamsAs1DForOutWhenUnconnected=off
  wires:
  Memory2/1 -> Triggered Subsystem1/1(In1)
  Product1/1 -> T/1, Memory2/1
  Pulse Generator1/1 -> Triggered Subsystem1/Trigger
  "Reset "/1 -> NOT1/1
  Triggered Subsystem1/1(Out1) -> Product1/1
  NOT1/1 -> Product1/2

== system pattern3x3_testing_2023v1/Neuron5/Subsystem2 ==
  note: 기존 membrane potential + input potential
  Input potential : Inport
  before_Potential : Inport  Port=2
  Trigger : TriggerPort  VariantControl=(inherit)  PortDimensions=1
  Sum : Sum  Inputs=|++
  membrane_state : Outport
  wires:
  Input potential/1 -> Sum/1
  Sum/1 -> membrane_state/1
  before_Potential/1 -> Sum/2

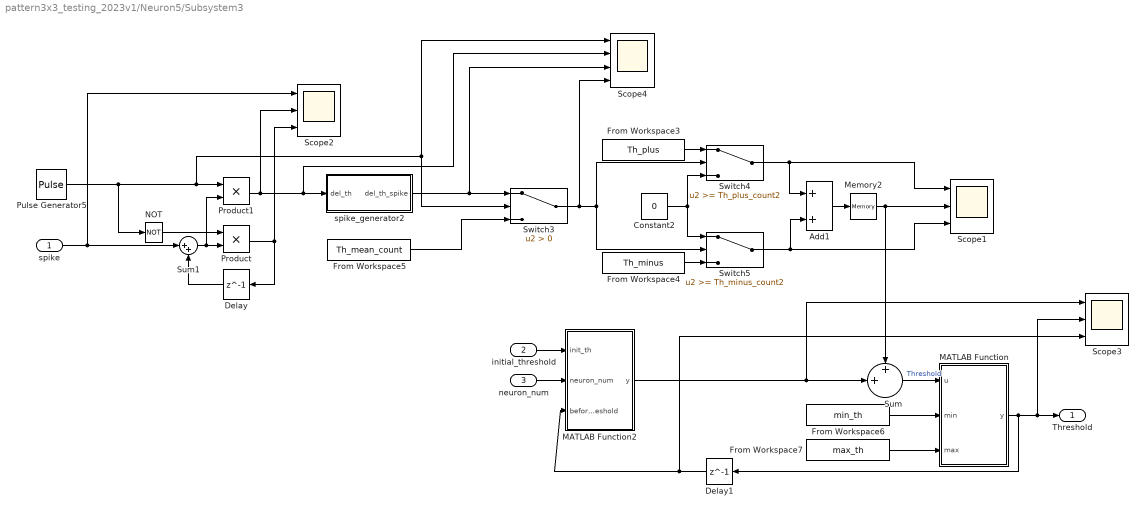
== system pattern3x3_testing_2023v1/Neuron5/Subsystem3 ==
  spike : Inport  OutDataTypeStr=double
  initial_threshold : Inport  Port=2
  neuron_num : Inport  Port=3
  Add1 : Sum
  Constant2 : Constant  Value=0
  Delay : Delay  DelayLength=1  SampleTime=0.00001
  Delay1 : Delay  DelayLength=1  SampleTime=0.00001
  From Workspace3 : FromWorkspace  VariableName=Th_plus
  From Workspace4 : FromWorkspace  VariableName=Th_minus
  From Workspace5 : FromWorkspace  VariableName=Th_mean_count
  From Workspace6 : FromWorkspace  VariableName=min_th
  From Workspace7 : FromWorkspace  VariableName=max_th
  MATLAB Function : MATLAB Function  TreatAsAtomicUnit=on
  MATLAB Function2 : MATLAB Function  TreatAsAtomicUnit=on
  Memory2 : Memory
  NOT : Logic  Operator=NOT  IconShape=distinctive  AllPortsSameDT=off  OutDataTypeStr=boolean
  Product : Product
  Product1 : Product
  Pulse Generator5 : DiscretePulseGenerator  PulseType=Time based  Period=Th_control_time2  PulseWidth=0.00001/Th_control_time2*100  PhaseDelay=Th_control_time2
  Scope1 : Scope  NumInputPorts=3
  Scope2 : Scope  NumInputPorts=3
  Scope3 : Scope  NumInputPorts=3
  Scope4 : Scope  NumInputPorts=4
  Sum : Sum  Inputs=++|
  Sum1 : Sum  Inputs=|++
  Switch3 : Switch  Criteria=u2 > Threshold  SaturateOnIntegerOverflow=off  InputSameDT=off
  Switch4 : Switch  Threshold=Th_plus_count2  SaturateOnIntegerOverflow=off  InputSameDT=off
  Switch5 : Switch  Threshold=Th_minus_count2  SaturateOnIntegerOverflow=off  InputSameDT=off
  spike_generator2 : Subsystem
  Threshold : Outport
  wires:
  MATLAB Function2/1(y) -> Scope3/1, Sum/2
  Sum/1 -> MATLAB Function/1(u)  "Threshold"
  From Workspace7/1 -> MATLAB Function/3(max)
  Delay1/1 -> Scope3/3, MATLAB Function2/3(before_threshold)
  neuron_num/1 -> MATLAB Function2/2(neuron_num)
  MATLAB Function/1(y) -> Delay1/1, Scope3/2, Threshold/1
  initial_threshold/1 -> MATLAB Function2/1(init_th)
  From Workspace6/1 -> MATLAB Function/2(min)
  Pulse Generator5/1 -> Switch3/2, Scope4/1, Product1/1, NOT/1
  Product1/1 -> Scope2/2, Scope4/2, spike_generator2/1(del_th)
  spike/1 -> Scope2/1, Sum1/1
  Delay/1 -> Sum1/2
  Product/1 -> Delay/1, Scope2/3
  Switch4/1 -> Add1/1, Scope1/1
  Switch5/1 -> Scope1/3, Add1/2
  Sum1/1 -> Product1/2, Product/2
  Constant2/1 -> Switch5/1, Switch4/3
  From Workspace4/1 -> Switch5/3
  Switch3/1 -> Scope4/4, Switch5/2, Switch4/2
  From Workspace3/1 -> Switch4/1
  NOT/1 -> Product/1
  spike_generator2/1(del_th_spike) -> Switch3/1, Scope4/3
  From Workspace5/1 -> Switch3/3
  Memory2/1 -> Scope1/2, Sum/1
  Add1/1 -> Memory2/1

== system pattern3x3_testing_2023v1/Neuron5/spike_generator1 ==
  1 : Inport
  AND : Logic  IconShape=distinctive  AllPortsSameDT=off  OutDataTypeStr=boolean
  Cast To Double : DataTypeConversion  OutDataTypeStr=double  SaturateOnIntegerOverflow=off  RndMeth=Floor
  Delay1 : Delay
  NOT : Logic  Operator=NOT  IconShape=distinctive  AllPortsSameDT=off  OutDataTypeStr=boolean
  Scope3 : Scope  NumInputPorts=5
  spike : Outport
  wires:
  NOT/1 -> Scope3/2, Delay1/1
  Delay1/1 -> Scope3/3, AND/2
  AND/1 -> Scope3/4, Cast To Double/1
  1/1 -> AND/1, Scope3/1, NOT/1
  Cast To Double/1 -> Scope3/5, spike/1

== system pattern3x3_testing_2023v1/Neuron6/Clock4 ==
  "Reset " : Inport
  Memory2 : Memory
  NOT1 : Logic  Operator=NOT  IconShape=distinctive  AllPortsSameDT=off  OutDataTypeStr=boolean
  Product1 : Product
  Pulse Generator1 : DiscretePulseGenerator  PulseType=Time based  Period=0.00001  PulseWidth=50
  Triggered Subsystem1 : Subsystem  TreatAsAtomicUnit=on
  T : Outport  VectorParamsAs1DForOutWhenUnconnected=off
  wires:
  Memory2/1 -> Triggered Subsystem1/1(In1)
  Product1/1 -> T/1, Memory2/1
  Pulse Generator1/1 -> Triggered Subsystem1/Trigger
  "Reset "/1 -> NOT1/1
  Triggered Subsystem1/1(Out1) -> Product1/1
  NOT1/1 -> Product1/2

== system pattern3x3_testing_2023v1/Neuron6/Clock5 ==
  "Reset " : Inport
  Memory2 : Memory
  NOT1 : Logic  Operator=NOT  IconShape=distinctive  AllPortsSameDT=off  OutDataTypeStr=boolean
  Product1 : Product
  Pulse Generator1 : DiscretePulseGenerator  PulseType=Time based  Period=0.00001  PulseWidth=50
  Triggered Subsystem1 : Subsystem  TreatAsAtomicUnit=on
  T : Outport  VectorParamsAs1DForOutWhenUnconnected=off
  wires:
  Memory2/1 -> Triggered Subsystem1/1(In1)
  Product1/1 -> T/1, Memory2/1
  Pulse Generator1/1 -> Triggered Subsystem1/Trigger
  "Reset "/1 -> NOT1/1
  Triggered Subsystem1/1(Out1) -> Product1/1
  NOT1/1 -> Product1/2

== system pattern3x3_testing_2023v1/Neuron6/Subsystem2 ==
  note: 기존 membrane potential + input potential
  Input potential : Inport
  before_Potential : Inport  Port=2
  Trigger : TriggerPort  VariantControl=(inherit)  PortDimensions=1
  Sum : Sum  Inputs=|++
  membrane_state : Outport
  wires:
  Input potential/1 -> Sum/1
  Sum/1 -> membrane_state/1
  before_Potential/1 -> Sum/2
